simulink model "Main_Simulink"  (R2023b)
settings: Solver=FixedStepDiscrete  StartTime=0.0  StopTime=inf  FixedStep=0.001  RelTol=1e-3
undefined symbols (not defined in the file or in its folder): battery_builder_rtmsupport, gcbh, Initial_SOC
libraries: nesl_utility x118, pack_105s34p_structured_lib x105, fl_lib x14, ee_lib x7, dspstat3 x6, BatteryBalancing x1, deeplib x1
(part 1 of 10)
settings Model: Creator=mcmas  LastModifiedBy=mcmas

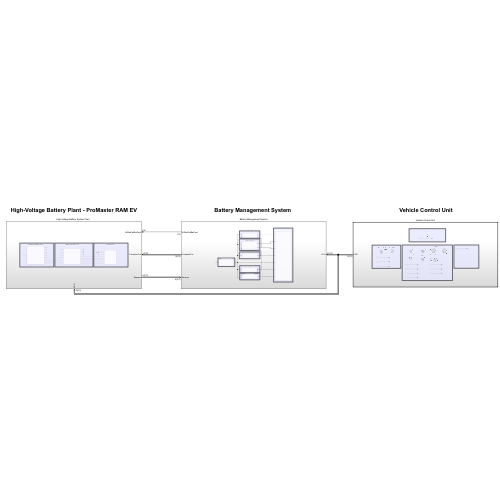
[thumbnail: Simulink's stored preview of the top-level diagram]
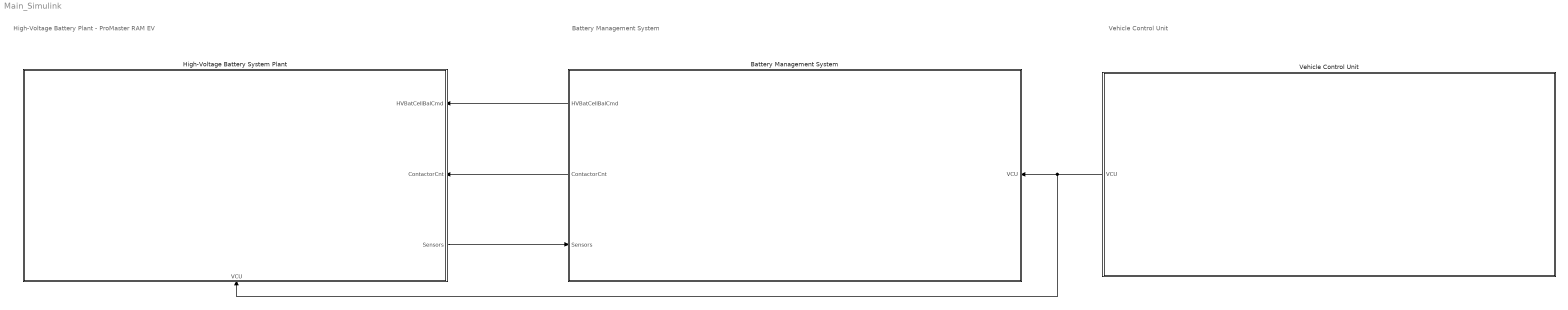
== system Main_Simulink ==
  note: High-Voltage Battery Plant - ProMaster RAM EV
  note: Battery Management System
  note: Vehicle Control Unit
  Battery Management System : Subsystem
      settings: PortSchema="{\"entries\":[{\"content\":{\"sides\":[{\"content\":{\"connectorIds\":[\"Out1\",\"Out2\",\"In1\"]},\"type\":\"ConnectorPlacement.EquallySpacedRectSide\",\"uuid\":\"9e8662b5-aff6-426b-8d2a-ef6b95784207\"},{\"content\":{\"connectorIds\":[\"In2\"],\"side\":\"RIGHT\"},\"type\":\"ConnectorPlacement.EquallySpacedRectSide\",\"uuid\":\"f4feacb2-8c13-4023-b441-c95415aec2f9\"},{\"content\":{\"side\":\"TOP\"},\"type\":\"ConnectorPlacement.EquallySpacedRectSide\",\"uuid\":\"0c24ddda-1492-4ea9-8759-203a1af902b3\"}]},\"type\":\"ConnectorPlacement.EquallySpacedConnector\",\"uuid\":\"40ebaec0-50fd-4c4b-bacf-e1435f1f9106\"}],\"packageUris\":[\"http://schema.mathworks.com/mf0/Connector/R2020b\"],\"version\":\"1.0\"}"
  "High-Voltage Battery System Plant   " : Subsystem  SystemSampleTime=0.001
      settings: PortSchema="{\"entries\":[{\"content\":{\"sides\":[{\"content\":{},\"type\":\"ConnectorPlacement.EquallySpacedRectSide\",\"uuid\":\"ae66c4d3-a535-4b5f-8246-6be0d2fba97c\"},{\"content\":{\"connectorIds\":[\"In2\",\"In3\",\"Out1\"],\"side\":\"RIGHT\"},\"type\":\"ConnectorPlacement.EquallySpacedRectSide\",\"uuid\":\"a52eeb25-f297-4e3b-9b18-4d751797d915\"},{\"content\":{\"side\":\"TOP\"},\"type\":\"ConnectorPlacement.EquallySpacedRectSide\",\"uuid\":\"98a0f19b-5094-4c94-9d4b-e54f955d4f3e\"},{\"content\":{\"connectorIds\":[\"In1\"],\"side\":\"BOTTOM\"},\"type\":\"ConnectorPlacement.EquallySpacedRectSide\",\"uuid\":\"dafcb442-8311-49ae-bfd4-efa25db882b8\"}]},\"type\":\"ConnectorPlacement.EquallySpacedConnector\",\"uuid\":\"e0e7d668-4082-4673-b7d0-0bd2f84fa0e5\"}],\"packageUris\":[\"http://schema.mathworks.com/mf0/Connector/R2020b\"],\"version\":\"1.0\"}"
  Vehicle Control Unit : Subsystem  TreatAsAtomicUnit=on  SystemSampleTime=0.001
  wires:
  Battery Management System/1(HVBatCellBalCmd) -> "High-Voltage Battery System Plant   "/2(HVBatCellBalCmd)
  "High-Voltage Battery System Plant   "/1(Sensors) -> Battery Management System/1(Sensors)
  Battery Management System/2(ContactorCnt) -> "High-Voltage Battery System Plant   "/3(ContactorCnt)
  Vehicle Control Unit/1(VCU) -> "High-Voltage Battery System Plant   "/1(VCU), Battery Management System/2(VCU)

== system Main_Simulink/Battery Management System ==
  note: Battery Monitoring System
  note: Fault Detection System
  note: Cell Balancing System
  note: State of Power System
  note: State of Charge System
  note: Contactor Drive System
  note: Communication Management System
  Sensors : Inport
  VCU : Inport  Port=2
  Battery Monitoring System : Subsystem
  Cell Balancing System : Subsystem
  Communication Management System : Subsystem
  Constant4 : Constant  Value=zeros(1,105)
  Contactor Drive System : Subsystem  TreatAsAtomicUnit=on  SystemSampleTime=0.001
  Fault Diagnosis System : Subsystem
  State of Charge Estimation System : Subsystem  TreatAsAtomicUnit=on  SystemSampleTime=1
  State of Power Estimation System : Subsystem  TreatAsAtomicUnit=on  SystemSampleTime=1
  HVBatCellBalCmd : Outport
  ContactorCnt : Outport  Port=2
  wires:
  Constant4/1 -> HVBatCellBalCmd/1
  Sensors/1 -> Battery Monitoring System/1(Sensors)
  Battery Monitoring System/1(BatteryMonitoringSystem) -> Cell Balancing System/1(BatteryMonitoringSystem), Contactor Drive System/2(BatteryMonitoringSystem), Fault Diagnosis System/1(BatteryMonitoringSystem), State of Power Estimation System/2(BatteryMonitoringSystem), State of Charge Estimation System/1(BatteryMonitoringSystem), Communication Management System/5(BatteryMonitoringSystem)
  State of Charge Estimation System/1(StateofChargeSystem) -> Contactor Drive System/3(StateofChargeSystem), Communication Management System/6(StateofChargeSystem), State of Power Estimation System/1(StateofChargeSystem)
  VCU/1 -> Contactor Drive System/1(VCU)
  Fault Diagnosis System/1(FaultDetectionSystem) -> Contactor Drive System/4(FaultDetectionSystem), Communication Management System/4(FaultDetectionSystem)
  Contactor Drive System/1(ContactorCnt) -> Communication Management System/2(ContactorCnt), ContactorCnt/1
  State of Power Estimation System/1(SystemofPowerSystem) -> Communication Management System/7(StateofPowerSystem)
  Cell Balancing System/1(HVBatCellBalCmd) -> Communication Management System/1(HVBatCellBalCmd)
  Contactor Drive System/2(PlugInCharging) -> Cell Balancing System/2(PlugInCharging), Communication Management System/3(PlugInCharging)

== system Main_Simulink/High-Voltage Battery System Plant    ==
  note: ProMaster EV Battery Pack
  note: Battery Disconnect Unit
  note: Charger/Load
  VCU : Inport
  HVBatCellBalCmd : Inport  Port=2
  Bus Element In2 : Inport  Port=3  PortName=ContactorCnt  Element=K1Main
  Bus Element In1 : Inport  Port=3  PortName=ContactorCnt  Element=K2Pre-
  Bus Element In3 : Inport  Port=3  PortName=ContactorCnt  Element=K3Pre+
  Bus Element In4 : Inport  Port=3  PortName=ContactorCnt  Element=K4DCFC
  "Battery Disconnect Unit " : Subsystem
  Bus Selector : BusSelector  OutputSignals=DCChargeCurrentReq,DrivingCurrentReq,ACChargeCurrentReq
  Charger/Load : Subsystem
  ProMaster EV Battery Pack : Subsystem
  Out Bus Element : Outport  PortName=Sensors  Element=HVBatteryVoltage_BEV
  Out Bus Element2 : Outport  PortName=Sensors  Element=HVBatCellVlt
  Out Bus Element3 : Outport  PortName=Sensors  Element=HVBatCellTemp
  Out Bus Element4 : Outport  PortName=Sensors  Element=HVBatClgInletTemp
  Out Bus Element5 : Outport  PortName=Sensors  Element=HVBatteryVoltage_BEV_DCFC
  Out Bus Element6 : Outport  PortName=Sensors  Element=HVBatteryVoltage_BEV_DCLink
  Out Bus Element8 : Outport  PortName=Sensors  Element=HVBatteryCurrent_BEV
  Out Bus Element1 : Outport  PortName=Sensors  Element=HVBatClgOutletTemp
  Out Bus Element7 : Outport  PortName=Sensors  Element=HVBatPrecharge_Temp
  wires:
  HVBatCellBalCmd/1 -> ProMaster EV Battery Pack/1(HVBatCellBalCmd)
  Bus Selector/1 -> Charger/Load/1(ChargeCurrentReq)  "<DCChargeCurrentReq>"
  Bus Selector/3 -> Charger/Load/3(ACChargeCurrentReq)  "<ACChargeCurrentReq>"
  ProMaster EV Battery Pack/1(HVBatteryVoltage_BEV) -> Out Bus Element/1
  ProMaster EV Battery Pack/2(HVBatCellVlt) -> Out Bus Element2/1  "HVBatCellVlt"
  ProMaster EV Battery Pack/3(HVBatCellTemp) -> Out Bus Element3/1
  ProMaster EV Battery Pack/4(HVBatClgInletTemp) -> Out Bus Element4/1
  "Battery Disconnect Unit "/1(HVBatPack_DCFCVoltage) -> Out Bus Element5/1
  "Battery Disconnect Unit "/2(HVBatteryVoltage_BEV_DCLink) -> Out Bus Element6/1
  "Battery Disconnect Unit "/3(HVBatteryCurrent_BEV) -> Out Bus Element8/1
  Bus Element In2/1 -> "Battery Disconnect Unit "/1(ContactorCnt_K1_Main)
  Bus Element In1/1 -> "Battery Disconnect Unit "/2(ContactorCnt_K2_Pre-)
  Bus Element In3/1 -> "Battery Disconnect Unit "/3(ContactorCnt_K3_Pre+)
  Bus Element In4/1 -> "Battery Disconnect Unit "/4(ContactorCnt_K4_DCFC)
  ProMaster EV Battery Pack/5(HVBatClgIOutletTemp) -> Out Bus Element1/1
  "Battery Disconnect Unit "/4(HVBatPrecharge_Temp) -> Out Bus Element7/1
  VCU/1 -> Bus Selector/1
  Bus Selector/2 -> Charger/Load/2(DrivingCurrentReq)  "<DrivingCurrentReq>"
  connections:
  ProMaster EV Battery Pack/RConn1 -- "Battery Disconnect Unit "/LConn1
  "Battery Disconnect Unit "/LConn2 -- ProMaster EV Battery Pack/RConn2
  "Battery Disconnect Unit "/RConn1 -- Charger/Load/LConn1
  "Battery Disconnect Unit "/RConn2 -- Charger/Load/LConn2
  "Battery Disconnect Unit "/RConn3 -- Charger/Load/LConn3
  "Battery Disconnect Unit "/RConn4 -- Charger/Load/LConn4
  "Battery Disconnect Unit "/RConn5 -- Charger/Load/LConn5

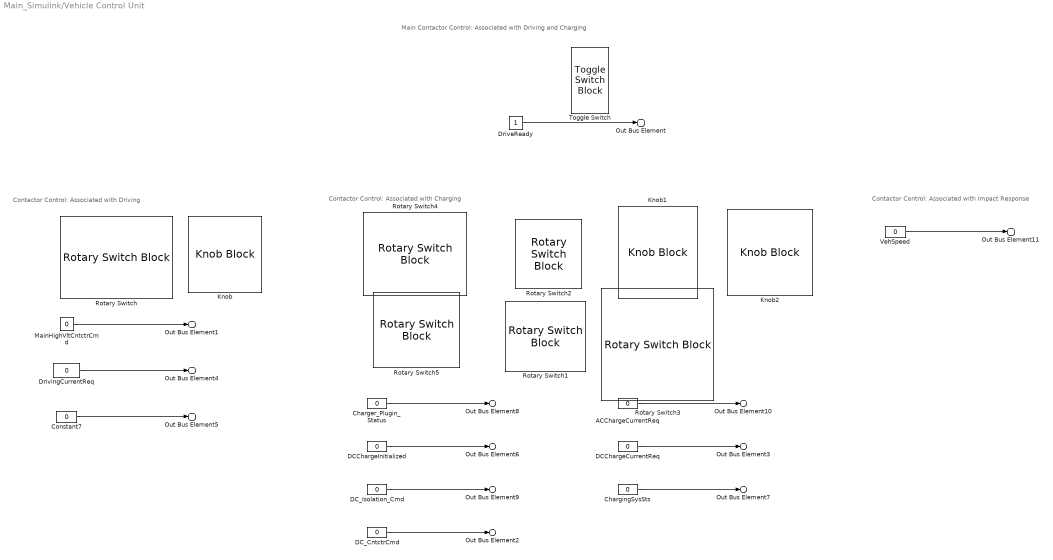
== system Main_Simulink/Vehicle Control Unit ==
  note: Main Contactor Control: Associated with Driving and Charging
  note: Contactor Control: Associated with Charging
  note: Contactor Control: Associated with Driving
  note: Contactor Control: Associated with Impact Response
  ACChargeCurrentReq : Constant  Value=0
  Charger_Plugin_Status : Constant  Value=0
  ChargingSysSts : Constant  Value=0
  Constant7 : Constant  Value=0
  DCChargeCurrentReq : Constant  Value=0
  DCChargeInitialized : Constant  Value=0
  DC_CntctrCmd : Constant  Value=0
  DC_Isolation_Cmd : Constant  Value=0
  DriveReady : Constant
  DrivingCurrentReq : Constant  Value=0
  Knob : KnobBlock  ScaleMax=322
  Knob1 : KnobBlock  ScaleMax=322
  Knob2 : KnobBlock
  MainHighVltCntctrCmd : Constant  Value=0
  Rotary Switch{,1..5} (6 alike) : RotarySwitchBlock
  Toggle Switch : ToggleSwitchBlock
      settings: Values={{'No', 'Yes'}, [0 1]}
  VehSpeed : Constant  Value=0
  Out Bus Element : Outport  PortName=VCU  Element=DriveReady
  Out Bus Element1 : Outport  PortName=VCU  Element=MainHighVltCntctrCmd
  Out Bus Element2 : Outport  PortName=VCU  Element=DC_CntctrCmd
  Out Bus Element3 : Outport  PortName=VCU  Element=DCChargeCurrentReq
  Out Bus Element4 : Outport  PortName=VCU  Element=DrivingCurrentReq
  Out Bus Element5 : Outport  PortName=VCU  Element=AccessoriesCurrentReq
  Out Bus Element6 : Outport  PortName=VCU  Element=DCChargeInitialized
  Out Bus Element7 : Outport  PortName=VCU  Element=ChargingSysSts
  Out Bus Element8 : Outport  PortName=VCU  Element=Charger_Plugin_Status
  Out Bus Element9 : Outport  PortName=VCU  Element=DC_Isolation_Cmd
  Out Bus Element10 : Outport  PortName=VCU  Element=ACChargeCurrentReq
  Out Bus Element11 : Outport  PortName=VCU  Element=VehSpeed
  wires:
  DC_CntctrCmd/1 -> Out Bus Element2/1
  MainHighVltCntctrCmd/1 -> Out Bus Element1/1
  DriveReady/1 -> Out Bus Element/1
  Constant7/1 -> Out Bus Element5/1
  DrivingCurrentReq/1 -> Out Bus Element4/1
  DCChargeCurrentReq/1 -> Out Bus Element3/1
  DCChargeInitialized/1 -> Out Bus Element6/1
  ChargingSysSts/1 -> Out Bus Element7/1
  Charger_Plugin_Status/1 -> Out Bus Element8/1
  DC_Isolation_Cmd/1 -> Out Bus Element9/1
  ACChargeCurrentReq/1 -> Out Bus Element10/1
  VehSpeed/1 -> Out Bus Element11/1

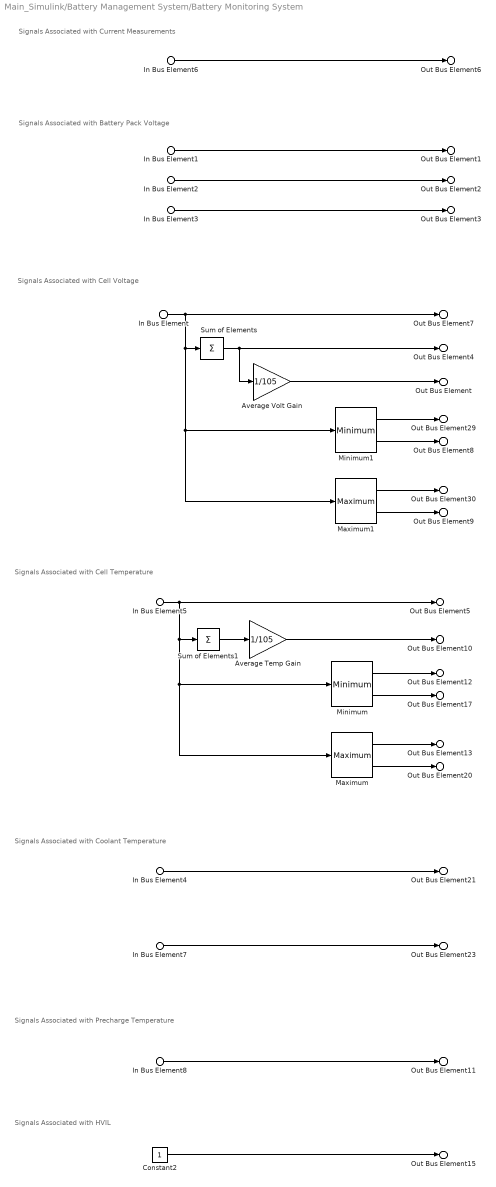
== system Main_Simulink/Battery Management System/Battery Monitoring System ==
  note: Signals Associated with HVIL
  note: Signals Associated with Coolant Temperature
  note: Signals Associated with Current Measurements
  note: Signals Associated with Battery Pack Voltage
  note: Signals Associated with Cell Temperature
  note: Signals Associated with Cell Voltage
  note: Signals Associated with Precharge Temperature
  In Bus Element : Inport  PortName=Sensors  Element=HVBatCellVlt
  In Bus Element1 : Inport  PortName=Sensors  Element=HVBatteryVoltage_BEV
  In Bus Element2 : Inport  PortName=Sensors  Element=HVBatteryVoltage_BEV_DCFC
  In Bus Element3 : Inport  PortName=Sensors  Element=HVBatteryVoltage_BEV_DCLink
  In Bus Element5 : Inport  PortName=Sensors  Element=HVBatCellTemp
  In Bus Element6 : Inport  PortName=Sensors  Element=HVBatteryCurrent_BEV
  In Bus Element4 : Inport  PortName=Sensors  Element=HVBatClgInletTemp
  In Bus Element7 : Inport  PortName=Sensors  Element=HVBatClgOutletTemp
  In Bus Element8 : Inport  PortName=Sensors  Element=HVBatPrecharge_Temp
  Average Temp Gain : Gain  Gain=1/105
  Average Volt Gain : Gain  Gain=1/105
  Constant2 : Constant
  Maximum : dspstat3/Maximum  operation=maximum  fcn=Value and Index  indexBase=One  operateOver=Each column  Dimension=1  InputProcessing=Columns as channels (frame based)  reset=None  roiEnable=off  roiType=Rectangles  roiPortion=Entire ROI  roiOutput=Individual statistics for each ROI  roiFlag=off  roundingMode=Floor  overflowMode=off  accumDataTypeStr=Inherit: Same as product output  accumLastDataTypeStr=Inherit: Same as product output
      settings: LibrarySourceBlock=dsphdlsupportstat/Maximum
  Maximum1 : dspstat3/Maximum  operation=maximum  fcn=Value and Index  indexBase=One  operateOver=Each column  Dimension=1  InputProcessing=Columns as channels (frame based)  reset=None  roiEnable=off  roiType=Rectangles  roiPortion=Entire ROI  roiOutput=Individual statistics for each ROI  roiFlag=off  roundingMode=Floor  overflowMode=off  accumDataTypeStr=Inherit: Same as product output  accumLastDataTypeStr=Inherit: Same as product output
      settings: LibrarySourceBlock=dsphdlsupportstat/Maximum
  Minimum : dspstat3/Minimum  operation=minimum  fcn=Value and Index  indexBase=One  operateOver=Each column  Dimension=1  InputProcessing=Columns as channels (frame based)  reset=None  roiEnable=off  roiType=Rectangles  roiPortion=Entire ROI  roiOutput=Individual statistics for each ROI  roiFlag=off  roundingMode=Floor  overflowMode=off
      settings: LibrarySourceBlock=dsphdlsupportstat/Minimum
  Minimum1 : dspstat3/Minimum  operation=minimum  fcn=Value and Index  indexBase=One  operateOver=Each column  Dimension=1  InputProcessing=Columns as channels (frame based)  reset=None  roiEnable=off  roiType=Rectangles  roiPortion=Entire ROI  roiOutput=Individual statistics for each ROI  roiFlag=off  roundingMode=Floor  overflowMode=off
      settings: LibrarySourceBlock=dsphdlsupportstat/Minimum
  Sum of Elements : Sum  Inputs=+
  Sum of Elements1 : Sum  Inputs=+
  Out Bus Element : Outport  PortName=BatteryMonitoringSystem  Element=HVBatCellVltAvg
  Out Bus Element1 : Outport  PortName=BatteryMonitoringSystem  Element=HVBatteryVoltage_BEV
  Out Bus Element2 : Outport  PortName=BatteryMonitoringSystem  Element=HVBatteryVoltage_BEV_DCFC
  Out Bus Element3 : Outport  PortName=BatteryMonitoringSystem  Element=HVBatteryVoltage_BEV_DCLink
  Out Bus Element5 : Outport  PortName=BatteryMonitoringSystem  Element=HVBatCellTemp
  Out Bus Element6 : Outport  PortName=BatteryMonitoringSystem  Element=HVBatteryCurrent_BEV
  Out Bus Element7 : Outport  PortName=BatteryMonitoringSystem  Element=HVBatCellVlt
  Out Bus Element4 : Outport  PortName=BatteryMonitoringSystem  Element=HVBatteryVoltage_BEV_Sec
  Out Bus Element8 : Outport  PortName=BatteryMonitoringSystem  Element=HVBatCellVlt_NumMin
  Out Bus Element9 : Outport  PortName=BatteryMonitoringSystem  Element=HVBatCellVlt_NumMax
  Out Bus Element10 : Outport  PortName=BatteryMonitoringSystem  Element=HVBatModTempAvg
  Out Bus Element12 : Outport  PortName=BatteryMonitoringSystem  Element=HVBatModTempMin
  Out Bus Element13 : Outport  PortName=BatteryMonitoringSystem  Element=HVBatModTempMax
  Out Bus Element17 : Outport  PortName=BatteryMonitoringSystem  Element=HVBatModTemp_NumMin
  Out Bus Element20 : Outport  PortName=BatteryMonitoringSystem  Element=HVBatModTemp_NumMax
  Out Bus Element21 : Outport  PortName=BatteryMonitoringSystem  Element=HVBatClgInletTemp
  Out Bus Element23 : Outport  PortName=BatteryMonitoringSystem  Element=HVBatClgOutletTemp
  Out Bus Element29 : Outport  PortName=BatteryMonitoringSystem  Element=HVBatCellVltMin
  Out Bus Element30 : Outport  PortName=BatteryMonitoringSystem  Element=HVBatCellVltMax
  Out Bus Element11 : Outport  PortName=BatteryMonitoringSystem  Element=HVBatPrecharge_Temp
  Out Bus Element15 : Outport  PortName=BatteryMonitoringSystem  Element=HVBatIntrlk_InternalStat
  wires:
  In Bus Element1/1 -> Out Bus Element1/1
  In Bus Element2/1 -> Out Bus Element2/1
  In Bus Element3/1 -> Out Bus Element3/1
  In Bus Element6/1 -> Out Bus Element6/1
  In Bus Element/1 -> Out Bus Element7/1, Minimum1/1, Maximum1/1, Sum of Elements/1
  Sum of Elements/1 -> Out Bus Element4/1, Average Volt Gain/1
  In Bus Element5/1 -> Maximum/1, Minimum/1, Sum of Elements1/1, Out Bus Element5/1
  Sum of Elements1/1 -> Average Temp Gain/1
  Average Temp Gain/1 -> Out Bus Element10/1
  Maximum/1 -> Out Bus Element13/1
  Minimum/1 -> Out Bus Element12/1
  Minimum/2 -> Out Bus Element17/1
  Maximum/2 -> Out Bus Element20/1
  In Bus Element4/1 -> Out Bus Element21/1
  In Bus Element7/1 -> Out Bus Element23/1
  Minimum1/2 -> Out Bus Element8/1
  Average Volt Gain/1 -> Out Bus Element/1
  Maximum1/2 -> Out Bus Element9/1
  Maximum1/1 -> Out Bus Element30/1
  Minimum1/1 -> Out Bus Element29/1
  In Bus Element8/1 -> Out Bus Element11/1
  Constant2/1 -> Out Bus Element15/1

== system Main_Simulink/Battery Management System/Cell Balancing System ==
  note: Battery Balancing Strategy
  In Bus Element : Inport  PortName=BatteryMonitoringSystem  Element=HVBatCellVlt
  In Bus Element1 : Inport  PortName=BatteryMonitoringSystem  Element=HVBatModTempMax
  In Bus Element2 : Inport  Port=2  PortName=PlugInCharging  Element=HVBatChargeStat
  Data Type Conversion : DataTypeConversion  OutDataTypeStr=double  SaturateOnIntegerOverflow=off  RndMeth=Floor
  MATLAB Function2 : MATLAB Function  TreatAsAtomicUnit=on
  MATLAB Function3 : MATLAB Function  TreatAsAtomicUnit=on
  Passive Cell Balancing : BatteryBalancing/Passive Cell Balancing  Threshold=0.01  HysteresisBand=0  Td_on=10  Td_off=60  Ts=-1  dataType=double
      settings: LibrarySourceBlock=batt_sl_lib/Cell Balancing/Passive Cell Balancing
  Unit Delay1 : UnitDelay  SampleTime=-1  HasFrameUpgradeWarning=on
  HVBatCellBalCmd : Outport
  HVBatCellBalStat : Outport  Port=2
  wires:
  In Bus Element/1 -> Passive Cell Balancing/1
  Passive Cell Balancing/2 -> MATLAB Function2/1(isBalancingActive_Curr)  "isBalancingActive"
  MATLAB Function3/1(BalancingEnabled) -> Passive Cell Balancing/2
  Passive Cell Balancing/1 -> Data Type Conversion/1
  Data Type Conversion/1 -> HVBatCellBalCmd/1
  MATLAB Function2/1(BalStat) -> HVBatCellBalStat/1, Unit Delay1/1
  Unit Delay1/1 -> MATLAB Function2/2(BalStat_Prev)
  In Bus Element1/1 -> MATLAB Function3/1(HVBatModTempMax)
  In Bus Element2/1 -> MATLAB Function3/2(HVBatChargeStat)

== system Main_Simulink/Battery Management System/Communication Management System ==
  note: CAN signals to be communicated to VCU
  HVBatCellBalCmd : Inport
  ContactorCnt : Inport  Port=2
  PlugInCharging : Inport  Port=3
  FaultDetectionSystem : Inport  Port=4
  BatteryMonitoringSystem : Inport  Port=5
  StateofChargeSystem : Inport  Port=6
  StateofPowerSystem : Inport  Port=7
  Bus Selector : BusSelector  OutputSignals=HVBatteryCurrent_BEV,HVBatteryVoltage_BEV,HVBatteryVoltage_BEV_DCLink,HVBatteryVoltage_BEV_DCFC,HVBatCellVltAvg,HVBatCellVltMin,HVBatCellVltMax,HVBatModTempAvg,HVBatModTempMin,HVBatModTempMax
  Bus Selector1 : BusSelector  OutputSignals=HVBatSOC,HVBatSOCMax,HVBatSOCMin
  Bus Selector2 : BusSelector  OutputSignals=HVBatDischrgPowInstant,HVBatDischrgPowShort,HVBatDischrgPowLong,HVBatDischrgPowCont,HVBatChrgPowInstant,HVBatChrgPowShort,HVBatChrgPowLong,HVBatChrgPowCont
  Bus Selector3 : BusSelector  OutputSignals=HVBatRdy,CellVltLow,CellVltHigh,ModTempLow,ModTempHigh
  Bus Selector4 : BusSelector  OutputSignals=K1Main,K2Pre-,K3Pre+,K4DCFC,HVBatCntctrStat
  Bus Selector5 : BusSelector  OutputSignals=DC_Isolation_Sts,HVBat_DC_CntctrStat,HVBatChargeStat,MaxChargeCurrentAllowed,HVBat_DC_CntctrOpn,HVBatCntctrReq,HVBatMaxCellVltAlld,HVBatMaxPkVltAllwd
  Mux{,1..3,7} (5 alike) : Mux  Inputs=3
  Mux4 : Mux  Inputs=8
  Mux5 : Mux  Inputs=5
  Mux6 : Mux
  Mux8 : Mux  Inputs=2
  Scope : Scope  NumInputPorts=12
  Terminator : Terminator
  Terminator1 : Terminator
  Terminator2 : Terminator
  wires:
  BatteryMonitoringSystem/1 -> Bus Selector/1
  Bus Selector/2 -> Mux/1  "<HVBatteryVoltage_BEV>"
  Bus Selector/3 -> Mux/2  "<HVBatteryVoltage_BEV_DCLink>"
  Bus Selector/4 -> Mux/3  "<HVBatteryVoltage_BEV_DCFC>"
  Bus Selector/5 -> Mux1/1  "<HVBatCellVltAvg>"
  Bus Selector/6 -> Mux1/2  "<HVBatCellVltMin>"
  Bus Selector/7 -> Mux1/3  "<HVBatCellVltMax>"
  Bus Selector/8 -> Mux2/1  "<HVBatModTempAvg>"
  Bus Selector/9 -> Mux2/2  "<HVBatModTempMin>"
  Bus Selector/10 -> Mux2/3  "<HVBatModTempMax>"
  StateofChargeSystem/1 -> Bus Selector1/1
  Bus Selector1/1 -> Mux3/1  "<HVBatSOC>"
  Bus Selector1/2 -> Mux3/2  "<HVBatSOCMax>"
  Bus Selector1/3 -> Mux3/3  "<HVBatSOCMin>"
  StateofPowerSystem/1 -> Bus Selector2/1
  Bus Selector2/1 -> Mux4/1  "<HVBatDischrgPowInstant>"
  Bus Selector2/2 -> Mux4/2  "<HVBatDischrgPowShort>"
  Bus Selector2/3 -> Mux4/3  "<HVBatDischrgPowLong>"
  Bus Selector2/4 -> Mux4/4  "<HVBatDischrgPowCont>"
  Bus Selector2/5 -> Mux4/5  "<HVBatChrgPowInstant>"
  Bus Selector2/8 -> Mux4/8  "<HVBatChrgPowCont>"
  Bus Selector2/7 -> Mux4/7  "<HVBatChrgPowLong>"
  Bus Selector2/6 -> Mux4/6  "<HVBatChrgPowShort>"
  FaultDetectionSystem/1 -> Bus Selector3/1
  Bus Selector3/3 -> Mux5/3  "<CellVltHigh>"
  Bus Selector3/2 -> Mux5/2  "<CellVltLow>"
  Bus Selector3/1 -> Mux5/1  "<HVBatRdy>"
  Bus Selector3/4 -> Mux5/4  "<ModTempLow>"
  Bus Selector3/5 -> Mux5/5  "<ModTempHigh>"
  Mux4/1 -> Scope/7
  Mux3/1 -> Scope/6
  Bus Selector/1 -> Scope/1  "<HVBatteryCurrent_BEV>"
  Mux/1 -> Scope/2
  Mux1/1 -> Scope/3
  Mux2/1 -> Scope/4
  Mux5/1 -> Scope/5
  ContactorCnt/1 -> Bus Selector4/1
  Bus Selector4/1 -> Mux6/1  "<K1Main>"
  Bus Selector4/2 -> Mux6/2  "<K2Pre->"
  Bus Selector4/3 -> Mux6/3  "<K3Pre+>"
  Bus Selector4/4 -> Mux6/4  "<K4DCFC>"
  Mux6/1 -> Scope/8
  Bus Selector4/5 -> Scope/9  "<HVBatCntctrStat>"
  PlugInCharging/1 -> Bus Selector5/1
  Bus Selector5/1 -> Mux7/1  "<DC_Isolation_Sts>"
  Bus Selector5/2 -> Mux7/2  "<HVBat_DC_CntctrStat>"
  Bus Selector5/3 -> Mux7/3  "<HVBatChargeStat>"
  Bus Selector5/5 -> Mux8/1  "<HVBat_DC_CntctrOpn>"
  Bus Selector5/6 -> Mux8/2  "<HVBatCntctrReq>"
  Mux7/1 -> Scope/10
  Mux8/1 -> Scope/11
  Bus Selector5/4 -> Scope/12  "<MaxChargeCurrentAllowed>"
  Bus Selector5/7 -> Terminator/1  "<HVBatMaxCellVltAlld>"
  Bus Selector5/8 -> Terminator1/1  "<HVBatMaxPkVltAllwd>"
  HVBatCellBalCmd/1 -> Terminator2/1

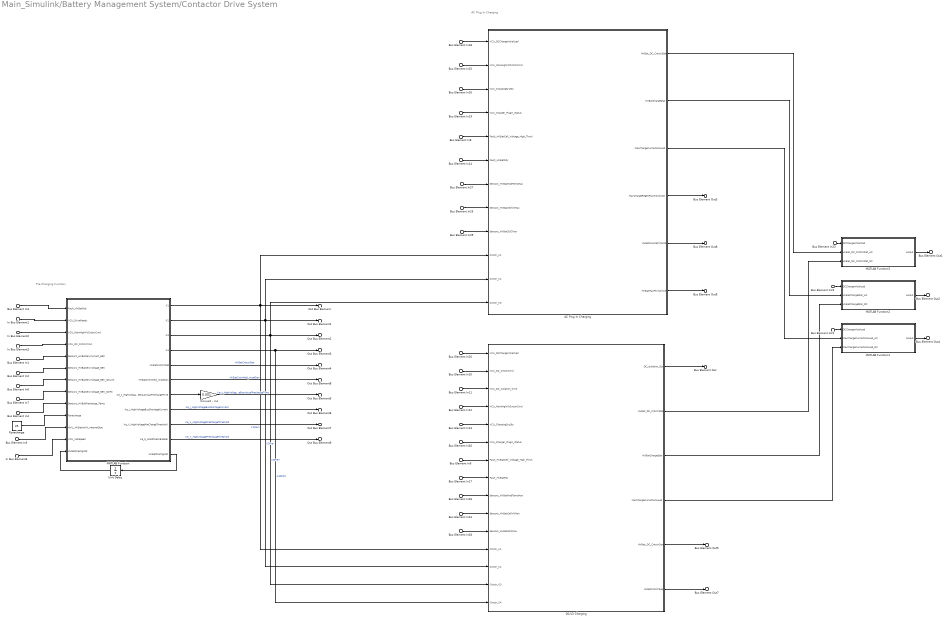
== system Main_Simulink/Battery Management System/Contactor Drive System ==
  note: AC Plug In Charging
  note: Pre-Charging Function
  In Bus Element1 : Inport  PortName=VCU  Element=DriveReady
  In Bus Element2 : Inport  PortName=VCU  Element=MainHighVltCntctrCmd
  Bus Element In12 : Inport  PortName=VCU  Element=MainHighVltCntctrCmd
  Bus Element In15 : Inport  PortName=VCU  Element=MainHighVltCntctrCmd
  In Bus Element3 : Inport  PortName=VCU  Element=DC_CntctrCmd
  Bus Element In10 : Inport  PortName=VCU  Element=DC_CntctrCmd
  Bus Element In11 : Inport  PortName=VCU  Element=DC_Isolation_Cmd
  Bus Element In13 : Inport  PortName=VCU  Element=ChargingSysSts
  Bus Element In16 : Inport  PortName=VCU  Element=ChargingSysSts
  Bus Element In{18,20..23} (5 alike) : Inport  PortName=VCU  Element=DCChargeInitialized
  Bus Element In19 : Inport  PortName=VCU  Element=Charger_Plugin_Status
  Bus Element In30 : Inport  PortName=VCU  Element=Charger_Plugin_Status
  In Bus Element4 : Inport  PortName=VCU  Element=VehSpeed
  Bus Element In2 : Inport  Port=2  PortName=BatteryMonitoringSystem  Element=HVBatteryVoltage_BEV
  Bus Element In1 : Inport  Port=2  PortName=BatteryMonitoringSystem  Element=HVBatteryCurrent_BEV
  Bus Element In6 : Inport  Port=2  PortName=BatteryMonitoringSystem  Element=HVBatteryVoltage_BEV_DCLink
  Bus Element In7 : Inport  Port=2  PortName=BatteryMonitoringSystem  Element=HVBatteryVoltage_BEV_DCFC
  Bus Element In4 : Inport  Port=2  PortName=BatteryMonitoringSystem  Element=HVBatPrecharge_Temp
  Bus Element In5 : Inport  Port=2  PortName=BatteryMonitoringSystem  Element=HVBatIntrlk_InternalStat
  Bus Element In24 : Inport  Port=2  PortName=BatteryMonitoringSystem  Element=HVBatCellVltMax
  Bus Element In25 : Inport  Port=2  PortName=BatteryMonitoringSystem  Element=HVBatCellVltMax
  Bus Element In26 : Inport  Port=2  PortName=BatteryMonitoringSystem  Element=HVBatModTempMax
  Bus Element In27 : Inport  Port=2  PortName=BatteryMonitoringSystem  Element=HVBatModTempMax
  Bus Element In28 : Inport  Port=3  PortName=StateofChargeSystem  Element=HVBatSOCMax
  Bus Element In29 : Inport  Port=3  PortName=StateofChargeSystem  Element=HVBatSOCMax
  Bus Element In3 : Inport  Port=4  PortName=FaultDetectionSystem  Element=HVBatRdy
  Bus Element In14 : Inport  Port=4  PortName=FaultDetectionSystem  Element=HVBatRdy
  Bus Element In17 : Inport  Port=4  PortName=FaultDetectionSystem  Element=HVBatRdy
  Bus Element In9 : Inport  Port=4  PortName=FaultDetectionSystem  Element=HVBatCell_Voltage_High_Thrsh
  Bus Element In8 : Inport  Port=4  PortName=FaultDetectionSystem  Element=HVBatCell_Voltage_High_Thrsh
  AC Plug In Charging : MATLAB Function  TreatAsAtomicUnit=on
  Convert - ms : Gain  Gain=0.001
  DC/L3 Charging : MATLAB Function  TreatAsAtomicUnit=on
  MATLAB Function : MATLAB Function  TreatAsAtomicUnit=on
  MATLAB Function1 : MATLAB Function  TreatAsAtomicUnit=on
  MATLAB Function2 : MATLAB Function  TreatAsAtomicUnit=on
  MATLAB Function3 : MATLAB Function  TreatAsAtomicUnit=on
  Rprecharge : Constant  Value=25
  Unit Delay : UnitDelay  SampleTime=-1  HasFrameUpgradeWarning=on
  Out Bus Element : Outport  PortName=ContactorCnt  Element=K1Main
  Out Bus Element1 : Outport  PortName=ContactorCnt  Element=K2Pre-
  Out Bus Element2 : Outport  PortName=ContactorCnt  Element=K3Pre+
  Out Bus Element3 : Outport  PortName=ContactorCnt  Element=K4DCFC
  Out Bus Element4 : Outport  PortName=ContactorCnt  Element=HVBatCntctrStat
  Out Bus Element5 : Outport  PortName=ContactorCnt  Element=Ke_t_HighVoltageBusActualPrechargeTime
  Out Bus Element6 : Outport  PortName=ContactorCnt  Element=Ke_I_HighVoltageBusShortageCurrent
  Out Bus Element7 : Outport  PortName=ContactorCnt  Element=Ke_V_HighVoltagePreChargeThreshold
  Out Bus Element8 : Outport  PortName=ContactorCnt  Element=HVBatCntrWeld_ImpdOpn
  Out Bus Element9 : Outport  PortName=ContactorCnt  Element=Ke_b_WeldCheckEnabler
  Bus Element Out : Outport  Port=2  PortName=PlugInCharging  Element=DC_Isolation_Sts
  Bus Element Out1 : Outport  Port=2  PortName=PlugInCharging  Element=HVBat_DC_CntctrStat
  Bus Element Out2 : Outport  Port=2  PortName=PlugInCharging  Element=HVBatChargeStat
  Bus Element Out3 : Outport  Port=2  PortName=PlugInCharging  Element=MaxChargeRegenPowerAllowed
  Bus Element Out4 : Outport  Port=2  PortName=PlugInCharging  Element=MaxChargeCurrentAllowed
  Bus Element Out5 : Outport  Port=2  PortName=PlugInCharging  Element=HVBat_DC_CntctrOpn
  Bus Element Out7 : Outport  Port=2  PortName=PlugInCharging  Element=HVBatCntctrReq
  Bus Element Out8 : Outport  Port=2  PortName=PlugInCharging  Element=HVBatMaxCellVltAlld
  Bus Element Out9 : Outport  Port=2  PortName=PlugInCharging  Element=HVBatMaxPkVltAllwd
  wires:
  Unit Delay/1 -> MATLAB Function/13("HVBatPrechgInbt ")
  In Bus Element3/1 -> MATLAB Function/4(VCU_DC_CntctrCmd)
  Bus Element In3/1 -> MATLAB Function/1(Fault_HVBatRdy)
  In Bus Element2/1 -> MATLAB Function/3(VCU_MainHighVltCntctrCmd)
  In Bus Element1/1 -> MATLAB Function/2(VCU_DriveReady)
  Bus Element In4/1 -> MATLAB Function/9(Sensors_HVBatPrecharge_Temp)
  Rprecharge/1 -> MATLAB Function/10(Rprecharge)
  Bus Element In5/1 -> MATLAB Function/11(HVIL_HVBatIntrlk_InternalStat)
  MATLAB Function/7(Ke_t_HighVoltageBusActualPrechargeTime) -> Convert - ms/1
  MATLAB Function/11(HVBatPrechgInbt) -> Unit Delay/1
  Bus Element In7/1 -> MATLAB Function/8(Sensors_HVBatteryVoltage_BEV_DCFC)
  MATLAB Function/9(Ke_V_HighVoltagePreChargeThreshold) -> Out Bus Element7/1  "Ke_V_HighVoltagePreChargeThreshold"
  MATLAB Function/5(HVBatCntctrStat) -> Out Bus Element4/1  "HVBatCntctrStat"
  MATLAB Function/3(K3) -> Out Bus Element2/1, DC/L3 Charging/14(Cntctr_K3), AC Plug In Charging/12(Cntctr_K3)  "K3Pre+"
  MATLAB Function/4(K4) -> Out Bus Element3/1, DC/L3 Charging/15(Cntctr_K4)  "K4DCFC"
  MATLAB Function/1(K1) -> Out Bus Element/1, DC/L3 Charging/12(Cntctr_K1), AC Plug In Charging/10(Cntctr_K1)  "K1Main"
  MATLAB Function/8(Ke_I_HighVoltageBusShortageCurrent) -> Out Bus Element6/1  "Ke_I_HighVoltageBusShortageCurrent"
  MATLAB Function/2(K2) -> Out Bus Element1/1, DC/L3 Charging/13(Cntctr_K2), AC Plug In Charging/11(Cntctr_K2)  "K2Pre-"
  Convert - ms/1 -> Out Bus Element5/1  "Ke_t_HighVoltageBusActualPrechargeTime"
  Bus Element In1/1 -> MATLAB Function/5(Sensors_HVBatteryCurrent_BEV)
  Bus Element In12/1 -> DC/L3 Charging/4(VCU_MainHighVltCntctrCmd)
  DC/L3 Charging/3(HVBatChargeStat) -> MATLAB Function2/3(HVBatChargeStat_DC)
  Bus Element In13/1 -> DC/L3 Charging/5(VCU_ChargingSysSts)
  Bus Element In25/1 -> AC Plug In Charging/8(Sensors_HVBatCellVltMax)
  DC/L3 Charging/2(HVBat_DC_CntctrStat) -> MATLAB Function3/3(HVBat_DC_CntctrStat_DC)
  Bus Element In8/1 -> AC Plug In Charging/5(Fault_HVBatCell_Voltage_High_Thrsh)
  Bus Element In11/1 -> DC/L3 Charging/3(VCU_DC_Isolation_Cmd)
  AC Plug In Charging/3(MaxChargeCurrentAllowed) -> MATLAB Function1/2(MaxChargeCurrentAllowed_AC)
  Bus Element In19/1 -> AC Plug In Charging/4(VCU_Charger_Plugin_Status)
  Bus Element In28/1 -> DC/L3 Charging/11(Sensors_HVBatSOCMax)
  AC Plug In Charging/6(HVBatMaxPkVltAllwd) -> Bus Element Out9/1
  MATLAB Function1/1(output) -> Bus Element Out4/1
  Bus Element In15/1 -> AC Plug In Charging/2(VCU_MainHighVltCntctrCmd)
  AC Plug In Charging/4(MaxChargeRegenPowerAllowed) -> Bus Element Out3/1
  Bus Element In16/1 -> AC Plug In Charging/3(VCU_ChargingSysSts)
  AC Plug In Charging/2(HVBatChargeStat) -> MATLAB Function2/2(HVBatChargeStat_AC)
  DC/L3 Charging/4(MaxChargeCurrentAllowed) -> MATLAB Function1/3(MaxChargeCurrentAllowed_DC)
  Bus Element In26/1 -> DC/L3 Charging/9(Sensors_HVBatModTempMax)
  Bus Element In29/1 -> AC Plug In Charging/9(Sensors_HVBatSOCMax)
  Bus Element In24/1 -> DC/L3 Charging/10(Sensors_HVBatCellVltMax)
  MATLAB Function2/1(output) -> Bus Element Out2/1
  MATLAB Function3/1(output) -> Bus Element Out1/1
  DC/L3 Charging/1(DC_Isolation_Sts) -> Bus Element Out/1
  Bus Element In27/1 -> AC Plug In Charging/7(Sensors_HVBatModTempMax)
  Bus Element In10/1 -> DC/L3 Charging/2(VCU_DC_CntctrCmd)
  Bus Element In17/1 -> DC/L3 Charging/8(Fault_HVBatRdy)
  DC/L3 Charging/6(HVBatCntctrReq) -> Bus Element Out7/1
  DC/L3 Charging/5(HVBat_DC_CntctrOpn) -> Bus Element Out5/1
  Bus Element In9/1 -> DC/L3 Charging/7(Fault_HVBatCell_Voltage_High_Thrsh)
  Bus Element In30/1 -> DC/L3 Charging/6(VCU_Charger_Plugin_Status)
  AC Plug In Charging/5(HVBatMaxCellVltAlld) -> Bus Element Out8/1
  AC Plug In Charging/1(HVBat_DC_CntctrStat) -> MATLAB Function3/2(HVBat_DC_CntctrStat_AC)
  Bus Element In14/1 -> AC Plug In Charging/6(Fault_HVBatRdy)
  Bus Element In18/1 -> AC Plug In Charging/1(VCU_DCChargeInitialized)
  Bus Element In20/1 -> DC/L3 Charging/1(VCU_DCChargeInitialized)
  Bus Element In21/1 -> MATLAB Function1/1(DCChargeInitialized)
  Bus Element In22/1 -> MATLAB Function2/1(DCChargeInitialized)
  Bus Element In23/1 -> MATLAB Function3/1(DCChargeInitialized)
  Bus Element In2/1 -> MATLAB Function/6(Sensors_HVBatteryVoltage_BEV)
  Bus Element In6/1 -> MATLAB Function/7(Sensors_HVBatteryVoltage_BEV_DCLink)
  MATLAB Function/6(HVBatCntrWeld_ImpdOpn) -> Out Bus Element8/1  "HVBatCntrWeld_ImpdOpn"
  MATLAB Function/10(Ke_b_WeldCheckEnabler) -> Out Bus Element9/1  "Ke_V_HighVoltagePreChargeThreshold"
  In Bus Element4/1 -> MATLAB Function/12(VCU_VehSpeed)

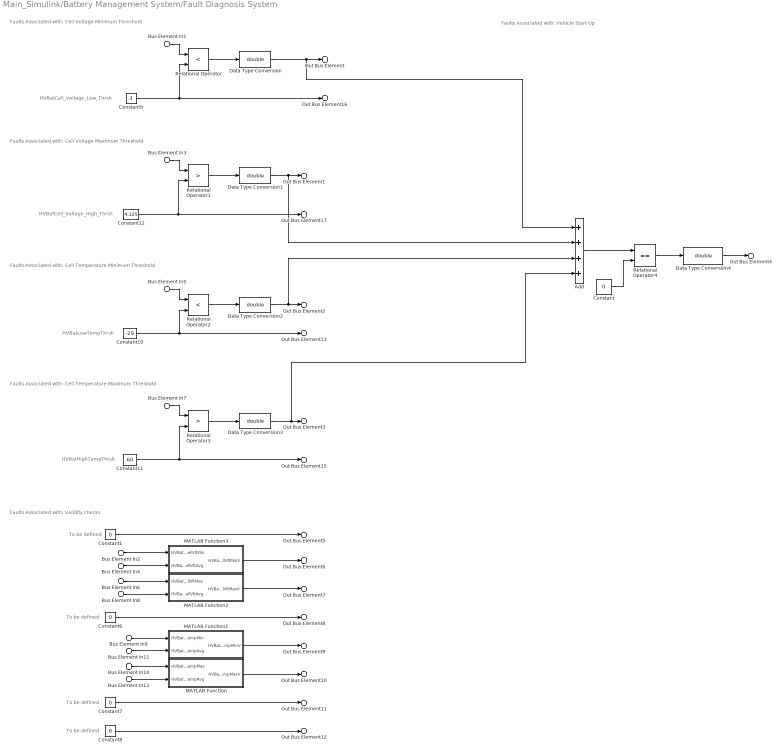
== system Main_Simulink/Battery Management System/Fault Diagnosis System ==
  note: Faults Associated with: Validity checks
  note: Faults Associated with: Vehicle Start-Up
  note: Faults Associated with: Cell Temperature Minimum Threshold
  note: Faults Associated with: Cell Voltage Maximum Threshold
  note: Faults Associated with: Cell Voltage Minimum Threshold
  note: Faults Associated with: Cell Temperature Maximum Threshold
  note: To be defined
  note: To be defined
  note: To be defined
  note: To be defined
  note: HVBatLowTempThrsh
  note: HVBatHighTempThrsh
  note: HVBatCell_Voltage_Low_Thrsh
  note: HVBatCell_Voltage_High_Thrsh
  Bus Element In1 : Inport  PortName=BatteryMonitoringSystem  Element=HVBatCellVltMin
  Bus Element In2 : Inport  PortName=BatteryMonitoringSystem  Element=HVBatCellVltMin
  Bus Element In3 : Inport  PortName=BatteryMonitoringSystem  Element=HVBatCellVltMax
  Bus Element In6 : Inport  PortName=BatteryMonitoringSystem  Element=HVBatCellVltMax
  Bus Element In5 : Inport  PortName=BatteryMonitoringSystem  Element=HVBatModTempMin
  Bus Element In9 : Inport  PortName=BatteryMonitoringSystem  Element=HVBatModTempMin
  Bus Element In7 : Inport  PortName=BatteryMonitoringSystem  Element=HVBatModTempMax
  Bus Element In10 : Inport  PortName=BatteryMonitoringSystem  Element=HVBatModTempMax
  Bus Element In4 : Inport  PortName=BatteryMonitoringSystem  Element=HVBatCellVltAvg
  Bus Element In8 : Inport  PortName=BatteryMonitoringSystem  Element=HVBatCellVltAvg
  Bus Element In11 : Inport  PortName=BatteryMonitoringSystem  Element=HVBatModTempAvg
  Bus Element In12 : Inport  PortName=BatteryMonitoringSystem  Element=HVBatModTempAvg
  Add : Sum  Inputs=++++
  Constant{,1,6..8} (5 alike) : Constant  Value=0
  Constant10 : Constant  Value=-29
  Constant11 : Constant  Value=60
  Constant12 : Constant  Value=4.125
  Constant9 : Constant  Value=3
  Data Type Conversion{,1..4} (5 alike) : DataTypeConversion  OutDataTypeStr=double  SaturateOnIntegerOverflow=off  RndMeth=Floor
  MATLAB Function : MATLAB Function  TreatAsAtomicUnit=on
  MATLAB Function1 : MATLAB Function  TreatAsAtomicUnit=on
  MATLAB Function2 : MATLAB Function  TreatAsAtomicUnit=on
  MATLAB Function3 : MATLAB Function  TreatAsAtomicUnit=on
  Relational Operator : RelationalOperator  Operator=<  OutDataTypeStr=boolean  RndMeth=Simplest  InputSameDT=off
  Relational Operator1 : RelationalOperator  Operator=>  OutDataTypeStr=boolean  RndMeth=Simplest  InputSameDT=off
  Relational Operator2 : RelationalOperator  Operator=<  OutDataTypeStr=boolean  RndMeth=Simplest  InputSameDT=off
  Relational Operator3 : RelationalOperator  Operator=>  OutDataTypeStr=boolean  RndMeth=Simplest  InputSameDT=off
  Relational Operator4 : RelationalOperator  Operator===  OutDataTypeStr=boolean  RndMeth=Simplest  InputSameDT=off
  Out Bus Element : Outport  PortName=FaultDetectionSystem  Element=CellVltLow
  Out Bus Element1 : Outport  PortName=FaultDetectionSystem  Element=CellVltHigh
  Out Bus Element2 : Outport  PortName=FaultDetectionSystem  Element=ModTempLow
  Out Bus Element3 : Outport  PortName=FaultDetectionSystem  Element=ModTempHigh
  Out Bus Element4 : Outport  PortName=FaultDetectionSystem  Element=HVBatRdy
  Out Bus Element5 : Outport  PortName=FaultDetectionSystem  Element=HVBatCellVltAvgV
  Out Bus Element6 : Outport  PortName=FaultDetectionSystem  Element=HVBatCellVltMinV
  Out Bus Element7 : Outport  PortName=FaultDetectionSystem  Element=HVBatCellVltMaxV
  Out Bus Element8 : Outport  PortName=FaultDetectionSystem  Element=HVBatModTempAvgV
  Out Bus Element9 : Outport  PortName=FaultDetectionSystem  Element=HVBatModTempMinV
  Out Bus Element10 : Outport  PortName=FaultDetectionSystem  Element=HVBatModTempMaxV
  Out Bus Element11 : Outport  PortName=FaultDetectionSystem  Element=HVBatClgOutletTempV
  Out Bus Element12 : Outport  PortName=FaultDetectionSystem  Element=HVBatClgInletTempV
  Out Bus Element13 : Outport  PortName=FaultDetectionSystem  Element=HVBatMod_Temperature_Low_Thrsh
  Out Bus Element15 : Outport  PortName=FaultDetectionSystem  Element=HVBatMod_Temperature_High_Thrsh
  Out Bus Element16 : Outport  PortName=FaultDetectionSystem  Element=HVBatCell_Voltage_Low_Thrsh
  Out Bus Element17 : Outport  PortName=FaultDetectionSystem  Element=HVBatCell_Voltage_High_Thrsh
  wires:
  Bus Element In1/1 -> Relational Operator/1
  Relational Operator/1 -> Data Type Conversion/1
  Data Type Conversion/1 -> Add/1, Out Bus Element/1
  Bus Element In3/1 -> Relational Operator1/1
  Relational Operator1/1 -> Data Type Conversion1/1
  Data Type Conversion1/1 -> Add/2, Out Bus Element1/1
  Data Type Conversion2/1 -> Add/3, Out Bus Element2/1
  Constant10/1 -> Relational Operator2/2, Out Bus Element13/1
  Relational Operator2/1 -> Data Type Conversion2/1
  Bus Element In5/1 -> Relational Operator2/1
  Data Type Conversion3/1 -> Add/4, Out Bus Element3/1
  Relational Operator3/1 -> Data Type Conversion3/1
  Bus Element In7/1 -> Relational Operator3/1
  Add/1 -> Relational Operator4/1
  Constant/1 -> Relational Operator4/2
  Relational Operator4/1 -> Data Type Conversion4/1
  MATLAB Function2/1(HVBatCellVltMaxV) -> Out Bus Element7/1
  MATLAB Function3/1(HVBatCellVltMinV) -> Out Bus Element6/1
  Constant1/1 -> Out Bus Element5/1
  MATLAB Function/1(HVBatModTempMaxV) -> Out Bus Element10/1
  Constant6/1 -> Out Bus Element8/1
  MATLAB Function1/1(HVBatModTempMinV) -> Out Bus Element9/1
  Constant7/1 -> Out Bus Element11/1
  Constant8/1 -> Out Bus Element12/1
  Constant11/1 -> Out Bus Element15/1, Relational Operator3/2
  Constant12/1 -> Relational Operator1/2, Out Bus Element17/1
  Constant9/1 -> Relational Operator/2, Out Bus Element16/1
  Data Type Conversion4/1 -> Out Bus Element4/1
  Bus Element In2/1 -> MATLAB Function3/1(HVBatCellVltMin)
  Bus Element In4/1 -> MATLAB Function3/2(HVBatCellVltAvg)
  Bus Element In6/1 -> MATLAB Function2/1(HVBatCellVltMax)
  Bus Element In8/1 -> MATLAB Function2/2(HVBatCellVltAvg)
  Bus Element In11/1 -> MATLAB Function1/2(HVBatModTempAvg)
  Bus Element In10/1 -> MATLAB Function/1(HVBatModTempMax)
  Bus Element In9/1 -> MATLAB Function1/1(HVBatModTempMin)
  Bus Element In12/1 -> MATLAB Function/2(HVBatModTempAvg)

== system Main_Simulink/Battery Management System/State of Charge Estimation System ==
  note: Pack-level SoC Estimator
  note: Cell-level SoC Estimator
  In Bus Element : Inport  PortName=BatteryMonitoringSystem  Element=HVBatCellVlt
  In Bus Element2 : Inport  PortName=BatteryMonitoringSystem  Element=HVBatCellTemp
  In Bus Element1 : Inport  PortName=BatteryMonitoringSystem  Element=HVBatteryCurrent_BEV
  Bus to Vector : BusToVector
  Bus to Vector1 : BusToVector
  Creating bus element : Subsystem
  For Each Subsystem1 : Subsystem  TreatAsAtomicUnit=on
  MATLAB Function : MATLAB Function  TreatAsAtomicUnit=on
  Maximum1 : dspstat3/Maximum  operation=maximum  fcn=Value and Index  indexBase=One  operateOver=Each column  Dimension=1  InputProcessing=Columns as channels (frame based)  reset=None  roiEnable=off  roiType=Rectangles  roiPortion=Entire ROI  roiOutput=Individual statistics for each ROI  roiFlag=off  roundingMode=Floor  overflowMode=off  accumDataTypeStr=Inherit: Same as product output  accumLastDataTypeStr=Inherit: Same as product output
      settings: LibrarySourceBlock=dsphdlsupportstat/Maximum
  Minimum1 : dspstat3/Minimum  operation=minimum  fcn=Value and Index  indexBase=One  operateOver=Each column  Dimension=1  InputProcessing=Columns as channels (frame based)  reset=None  roiEnable=off  roiType=Rectangles  roiPortion=Entire ROI  roiOutput=Individual statistics for each ROI  roiFlag=off  roundingMode=Floor  overflowMode=off
      settings: LibrarySourceBlock=dsphdlsupportstat/Minimum
  Pack-to-Cell (Scaling) : Gain  Gain=1/34
  Selector1 : Selector  InputPortWidth=105  IndexOptions=Index vector (dialog)  Indices=[1:105]  OutputSizes=1
  Selector210 : Selector  InputPortWidth=105  IndexOptions=Index vector (dialog)  Indices=[1:105]  OutputSizes=1
  Out Bus Element : Outport  PortName=StateofChargeSystem  Element=HVBatSOCMax
  Out Bus Element1 : Outport  PortName=StateofChargeSystem  Element=HVBatSOCMin
  Out Bus Element2 : Outport  PortName=StateofChargeSystem  Element=HVBatSOC_NumMin
  Out Bus Element3 : Outport  PortName=StateofChargeSystem  Element=HVBatSOC_NumMax
  Out Bus Element4 : Outport  PortName=StateofChargeSystem  Element=HVBatSOC
  wires:
  In Bus Element1/1 -> Pack-to-Cell (Scaling)/1
  In Bus Element2/1 -> Selector1/1
  In Bus Element/1 -> Selector210/1
  Pack-to-Cell (Scaling)/1 -> For Each Subsystem1/1(HVBatteryCurrent_BEV)
  Minimum1/1 -> MATLAB Function/1(MinCellSOC), Out Bus Element1/1
  Minimum1/2 -> Out Bus Element2/1
  Maximum1/1 -> MATLAB Function/2(MaxCellSOC), Out Bus Element/1
  Maximum1/2 -> Out Bus Element3/1
  Selector210/1 -> Bus to Vector/1
  Bus to Vector1/1 -> For Each Subsystem1/3(HVBatCellTemp)
  Bus to Vector/1 -> For Each Subsystem1/2(HVBatCellVlt)
  For Each Subsystem1/1(HvBatSOCcell) -> Creating bus element/1(HvBatSOCcell)
  Creating bus element/1(HVBatSOCcell) -> Minimum1/1, Maximum1/1
  Selector1/1 -> Bus to Vector1/1
  MATLAB Function/1(HVBatSOC) -> Out Bus Element4/1

== system Main_Simulink/Battery Management System/State of Power Estimation System ==
  note: Continuous Power Limits - Rolling Window Strategy
  note: Static Power Limits
  note: Continuous Charge Power Limits
  note: Continuous Discharge Power Limits
  note: Charge Power Limits
  note: Discharge Power Limits
  Bus Element In1 : Inport  PortName=StateofChargeSystem  Element=HVBatSOCMax
  Bus Element In2 : Inport  PortName=StateofChargeSystem  Element=HVBatSOCMin
  Bus Element In3 : Inport  Port=2  PortName=BatteryMonitoringSystem  Element=HVBatModTempMax
  Bus Element In4 : Inport  Port=2  PortName=BatteryMonitoringSystem  Element=HVBatModTempMin
  Bus Element In5 : Inport  Port=2  PortName=BatteryMonitoringSystem  Element=HVBatteryCurrent_BEV
  Bus Element In6 : Inport  Port=2  PortName=BatteryMonitoringSystem  Element=HVBatteryVoltage_BEV_Sec
  Bus Creator : BusCreator  Inputs=2
  Bus Creator2 : BusCreator  Inputs=4
  Bus Selector : BusSelector  OutputSignals=HVBatModTempMin,HVBatModTempMax,HVBatSOCMin
  Bus Selector1 : BusSelector  OutputSignals=HVBatModTempMin,HVBatModTempMax,HVBatSOCMax
  Continuus Charge Power Limits : Subsystem
  Continuus Discharge Power Limits : Subsystem
  Maximum Charge Power Limits : Subsystem
  Maximum Discharge Power Limits : Subsystem  SystemSampleTime=1
  Bus Element Out : Outport  PortName=SystemofPowerSystem  Element=HVBatDischrgPowInstant
  Bus Element Out1 : Outport  PortName=SystemofPowerSystem  Element=HVBatDischrgPowShort
  Bus Element Out2 : Outport  PortName=SystemofPowerSystem  Element=HVBatDischrgPowLong
  Bus Element Out3 : Outport  PortName=SystemofPowerSystem  Element=HVBatDischrgPowCont
  Bus Element Out4 : Outport  PortName=SystemofPowerSystem  Element=HVBatChrgPowInstant
  Bus Element Out5 : Outport  PortName=SystemofPowerSystem  Element=HVBatChrgPowShort
  Bus Element Out6 : Outport  PortName=SystemofPowerSystem  Element=HVBatChrgPowLong
  Bus Element Out7 : Outport  PortName=SystemofPowerSystem  Element=HVBatChrgPowCont
  wires:
  Bus Creator2/1 -> Bus Selector/1, Bus Selector1/1
  Bus Element In5/1 -> Bus Creator/1
  Bus Element In6/1 -> Bus Creator/2
  Continuus Discharge Power Limits/3(BPCM_HVBatDischrgPowLong) -> Bus Element Out2/1
  Continuus Discharge Power Limits/4(BPCM_HVBatDischrgPowCont) -> Bus Element Out3/1
  Maximum Discharge Power Limits/1(MaxPowertDischg) -> Continuus Discharge Power Limits/2(MaxPowerDisch)
  Bus Creator/1 -> Continuus Discharge Power Limits/1(BatteryMonitoringSystem), Continuus Charge Power Limits/1(BatteryMonitoringSystem)
  Bus Selector/2 -> Maximum Discharge Power Limits/2(HVBatModTempMax)  "<HVBatModTempMax>"
  Maximum Charge Power Limits/1(MaxPowerChrg) -> Continuus Charge Power Limits/2(MaxPowerChrg)
  Bus Selector/1 -> Maximum Discharge Power Limits/1(HVBatModTempMin)  "<HVBatModTempMin>"
  Bus Selector/3 -> Maximum Discharge Power Limits/3(HVBatSOCMin)  "<HVBatSOCMin>"
  Bus Selector1/3 -> Maximum Charge Power Limits/3(HVBatSOCMin)  "<HVBatSOCMax>"
  Bus Selector1/2 -> Maximum Charge Power Limits/2(HVBatModTempMax)  "<HVBatModTempMax>"
  Bus Selector1/1 -> Maximum Charge Power Limits/1(HVBatModTempMin)  "<HVBatModTempMin>"
  Continuus Discharge Power Limits/1(BPCM_HVBatDischrgPowInstant) -> Bus Element Out/1
  Bus Element In1/1 -> Bus Creator2/3
  Bus Element In2/1 -> Bus Creator2/4
  Bus Element In3/1 -> Bus Creator2/1
  Bus Element In4/1 -> Bus Creator2/2
  Continuus Discharge Power Limits/2(BPCM_HVBatDischrgPowShort) -> Bus Element Out1/1
  Continuus Charge Power Limits/3(BPCM_HVBatChrgPowLong) -> Bus Element Out6/1
  Continuus Charge Power Limits/4(BPCM_HVBatChrgPowCont) -> Bus Element Out7/1
  Continuus Charge Power Limits/1(BPCM_HVBatChrgPowInstant) -> Bus Element Out4/1
  Continuus Charge Power Limits/2(BPCM_HVBatChrgPowShort) -> Bus Element Out5/1
